simulink model "HeteroMK"  (R2020a)
settings: Solver=FixedStepAuto  StartTime=0.0  StopTime=10.0  RelTol=1e-3
libraries: simulink x1
settings Model: Creator=sadamu  LastModifiedBy=sadamu
settings OptimizationCC: OptimizeBlockIOStorage=off  OptimizeDataStoreBuffers=off  BusAssignmentInplaceUpdate=off
settings DebuggingCC: SFUnexpectedBacktrackingDiag=warning  SFNoUnconditionalDefaultTransitionDiag=warning
settings RTWCC: GenerateReport=on  BuildConfiguration=Debug  LaunchReport=on
settings CodeAppCC: ForceParamTrailComments=on  GenerateComments=off  MATLABSourceComments=on  EnableCustomComments=on
settings GRTTargetCC: CombineSignalStateStructs=on  SupportVariableSizeSignals=on  MultiInstanceErrorCode=Warning

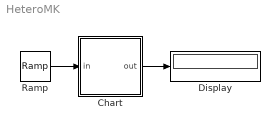
== system HeteroMK ==
  Chart : Stateflow chart  TreatAsAtomicUnit=on
  Display : Display
  Ramp : simulink/Sources/Ramp  slope=1  start=0  InitialOutput=0
  wires:
  Ramp/1 -> Chart/1(in)
  Chart/1(out) -> Display/1

== stateflow chart HeteroMK/Chart ==
  settings: updateMethod=DISCRETE  sampleTime=1
  state State1
    out = in
  state State2
    out = -in
  (default) -> State1
  State1 -> State2 : [mod(in,3)==0]
  State2 -> State1 : [mod(in,2)==0]
  data: in input; out output
